simulink model "controldesign_virt"  (Simulink 6.3)
settings: Solver=ode45  StartTime=0.0  StopTime=3  RelTol=1e-3
StopFcn:
  | save_system(vars.simfilename);
libraries: simulink x1, simulink_extras x1
CloseFcn:
  | save_system(vars.simfilename); sim(vars.simfilename);vars.simtime = str2num(get_param(vars.simfilename,'StopTime'));set(guiel.hSimtime,'String',num2str(vars.simtime));if strcmp(vars.simfilename(end-2:end),'sim') vars.L= motorParams(1,1); vars.R= motorParams(1,2); vars.J= motorParams(1,3);vars.b= motorParams(1,4); vars.Kb= motorParams(1,5); vars.Km= motorParams(1,6);if (min(size(motorParams)) == 9) vars.P= motorParams(1,7); vars.I= motorParams(1,8); vars.D= motorParams(1,9);else;vars.P= NaN; vars.I= NaN; vars.D= NaN;end;clear motorParams; [vars.numericTF vars.symbolTF] = calcTF2(vars);end,
settings Model: LastModifiedBy=michael  StrictBusMsg=None
settings DataIOCC: MaxDataPoints=10000
settings OptimizationCC: BlockReduction=off  BooleanDataType=off
settings DebuggingCC: SolverPrmCheckMsg=none
settings HardwareCC: TargetUnknown=on

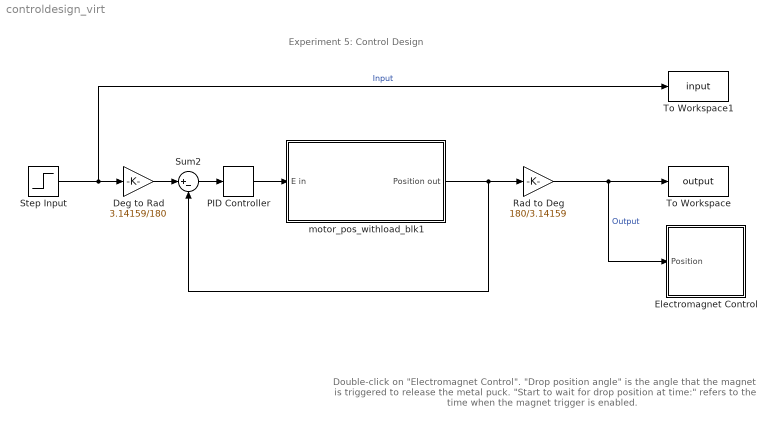
== system controldesign_virt ==
  note: Experiment 5: Control Design
  note: Double-click on "Electromagnet Control".
      |
      | "Drop position angle" is the angle that the
      | magnet is triggered to release the metal puck.
      |
      | "Start to wait for drop position at time:"
      | refers to the time when the magnet trigger is
      | enabled.
  Deg to Rad : Gain  Gain=3.14159/180  SaturateOnIntegerOverflow=on
  Electromagnet Control : Subsystem  mask{DropAngle=-500, Wait=1.6}
      mask prompts: DropAngle "Drop position angle"; Wait "Start to wait for drop position at time:"
  PID Controller : simulink_extras/Additional Linear/PID Controller  P=68  I=0  D=.1
  Rad to Deg : Gain  Gain=180/3.14159  SaturateOnIntegerOverflow=on
  Step Input : Step  Time=0.5  After=-500  SampleTime=0
  Sum2 : Sum  Inputs=|+-  SaturateOnIntegerOverflow=on  InputSameDT=on
  To Workspace : ToWorkspace  VariableName=output  SampleTime=-1  SaveFormat=Structure With Time
  To Workspace1 : ToWorkspace  VariableName=input  SampleTime=-1  SaveFormat=Structure With Time
  motor_pos_withload_blk1 : Subsystem
      mask Description: Real-Time Workshop generated S-function.
      mask Help: web(['file://',docroot,'/toolbox/rtw/rtwsfcn.html']);
      mask Display: disp('DC Motor (Position Control)')
  wires:
  Rad to Deg/1 -> To Workspace/1, Electromagnet Control/1(Position)  "Output"
  motor_pos_withload_blk1/1(Position out) -> Sum2/2, Rad to Deg/1
  PID Controller/1 -> motor_pos_withload_blk1/1(E in)
  Sum2/1 -> PID Controller/1
  Deg to Rad/1 -> Sum2/1
  Step Input/1 -> Deg to Rad/1, To Workspace1/1  "Input"

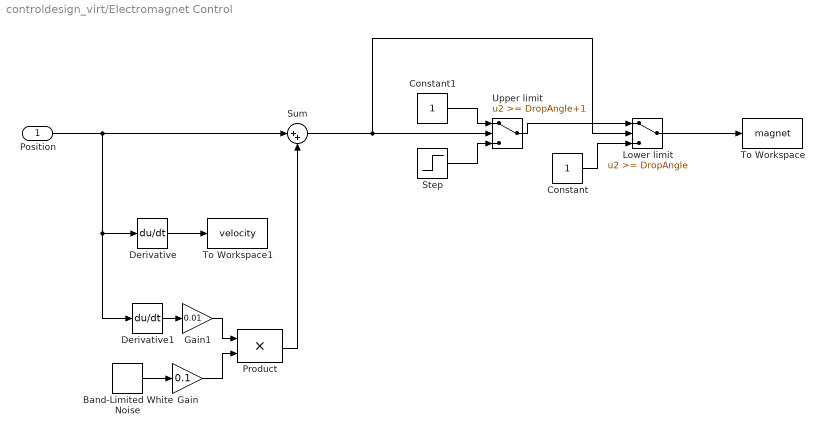
== system controldesign_virt/Electromagnet Control ==
  Position : Inport
  Band-Limited White Noise : simulink/Sources/Band-Limited White Noise  Cov=[0.01]  Ts=0.01  seed=[23341]
  Constant : Constant
  Constant1 : Constant
  Derivative : Derivative
  Derivative1 : Derivative
  Gain : Gain  Gain=0.1  SaturateOnIntegerOverflow=on
  Gain1 : Gain  Gain=0.01  SaturateOnIntegerOverflow=on
  Lower limit : Switch  Threshold=DropAngle  SaturateOnIntegerOverflow=on  InputSameDT=on
  Product : Product  SaturateOnIntegerOverflow=on  RndMeth=Zero  InputSameDT=on
  Step : Step  Time=Wait  Before=1  After=0  SampleTime=0
  Sum : Sum  Inputs=|++  SaturateOnIntegerOverflow=on  InputSameDT=on
  To Workspace : ToWorkspace  VariableName=magnet  SampleTime=-1  SaveFormat=Structure With Time
  To Workspace1 : ToWorkspace  VariableName=velocity  SampleTime=-1  SaveFormat=Structure With Time
  Upper limit : Switch  Threshold=DropAngle+1  SaturateOnIntegerOverflow=on  InputSameDT=on
  wires:
  Position/1 -> Sum/1, Derivative/1, Derivative1/1
  Step/1 -> Upper limit/3
  Constant1/1 -> Upper limit/1
  Constant/1 -> Lower limit/3
  Upper limit/1 -> Lower limit/1
  Lower limit/1 -> To Workspace/1
  Derivative/1 -> To Workspace1/1
  Derivative1/1 -> Gain1/1
  Band-Limited White Noise/1 -> Gain/1
  Gain/1 -> Product/2
  Product/1 -> Sum/2
  Gain1/1 -> Product/1
  Sum/1 -> Upper limit/2, Lower limit/2

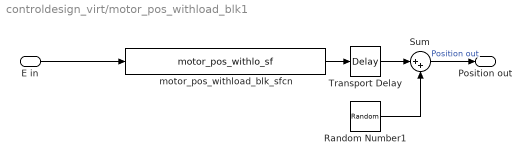
== system controldesign_virt/motor_pos_withload_blk1 ==
  E in : Inport
  Random Number1 : RandomNumber  Variance=0.000005  SampleTime=0.005
  Sum : Sum  Inputs=|++  SaturateOnIntegerOverflow=on  InputSameDT=on
  Transport Delay : TransportDelay  DelayTime=0.001  BufferSize=10000
  motor_pos_withload_blk_sfcn : S-Function  FunctionName=motor_pos_withlo_sf  SFunctionModules=""  mask{rtw_sf_name=motor_pos_withlo_sf, showVar=off}
      mask prompts: rtw_sf_name "Generated S-function name (model_sf):"; showVar "Show module list"
      mask help: Real-Time Workshop generated S-function.
      mask init:
      | displist = '';
      | if ~strcmp(get_param(gcb, 'FunctionName'), rtw_sf_name);
      |   set_param(gcb, 'FunctionName', rtw_sf_name);
      | end
      | if  showVar & exist('rtwsfunc') == 2
      |   tmplist = rtwsfunc(rtw_sf_name,gcb);
      |   tmplist = ['\nList of Modules:\n', tmplist];
      | elseif showVar
      |   tmplist = '\nList of Modules:\nRTW not licensed\n';
      | end
      | if showVar
      |   displist = tmplist;
      | end
      settings: CopyFcn=set_param(gcb,'linkstatus','none')
      mask Help: web(['file://',docroot,'/toolbox/rtw/rtwsfcn.html']);
      mask Display:
      | port_label('input',1,'E in');
      | port_label('output',1,'Position out');
  Position out : Outport
  wires:
  motor_pos_withload_blk_sfcn/1 -> Transport Delay/1
  Random Number1/1 -> Sum/2
  Transport Delay/1 -> Sum/1
  E in/1 -> motor_pos_withload_blk_sfcn/1
  Sum/1 -> Position out/1  "Position out"
